simulink model "encoder_slsp"  (Simulink 8.0)
settings: Solver=FixedStepDiscrete  SolverMode=SingleTasking  StartTime=0.0  StopTime=10.0  RelTol=1e-3
settings Model: Creator=gcampa  LastModifiedBy=gcampa  ExtModeTrigDuration=2
settings DataIOCC: SignalLoggingSaveFormat=ModelDataLogs  SaveOutput=off  SaveTime=off
settings OptimizationCC: OptimizeModelRefInitCode=on  LifeSpan=1
settings DebuggingCC: SolverPrmCheckMsg=none  FcnCallInpInsideContextMsg=EnableAllAsWarning  StrictBusMsg=Warning
settings HardwareCC: ProdBitPerInt=16  ProdBitPerPointer=16  ProdIntDivRoundTo=Zero  ProdEndianess=LittleEndian  ProdWordSize=8  ProdHWDeviceType=Atmel->AVR
settings RTWCC: SystemTargetFile=realtime.tlc  GenerateMakefile=off  TemplateMakefile=realtime.tmf  Description=Real-Time Toolbox  RTWVerbose=off  ProcessScript=realtime_make_rtw_hook
settings STFCustomTargetCC: TargetLibSuffix=.a  CodeReplacementLibrary=ANSI_C  GenerateSampleERTMain=on  ERTCustomFileBanners=on  SupportNonInlinedSFcns=off  SupportVariableSizeSignals=on  GRTInterface=off  SystemTargetFile=realtime.tlc
settings ERTTargetCC: CodeReplacementLibrary=ANSI_C  MultiwordLength=2048  GenerateSampleERTMain=on  ParMdlRefBuildCompliant=off  CompOptLevelCompliant=off  ConcurrentExecutionCompliant=off  CombineOutputUpdateFcns=off  ERTFirstTimeCompliant=off  SupportContinuousTime=on  SupportVariableSizeSignals=on  ModelStepFunctionPrototypeControlCompliant=off  CPPClassGenCompliant=off  ExtModeTransport=3  ExtModeMexFile=ext_serial_win32_comm  ExtModeMexArgs=0 1 9600  InlinedParameterPlacement=NonHierarchical  ERTSrcFileBannerTemplate=realtime_code_template.cgt  ERTHdrFileBannerTemplate=realtime_code_template.cgt  ERTDataSrcFileTemplate=realtime_code_template.cgt  ERTDataHdrFileTemplate=realtime_code_template.cgt  ERTCustomFileTemplate=realtime_file_process.tlc  ConvertIfToSwitch=off  SuppressUnreachableDefaultCases=off
settings SettingsController: Description=Run on Hardware Dialog  TargetExtensionPlatform=Arduino Uno
settings MATStruct: Set_host_COM_port=[0.0]  COM_port_number=1  COM_port_baud_rate=115200  Enable_overrun_detection=[0.0]  Digital_output_to_set_on_overrun=13  Analog_input_reference_voltage=[0.0]  Serial0_baud_rate=115200

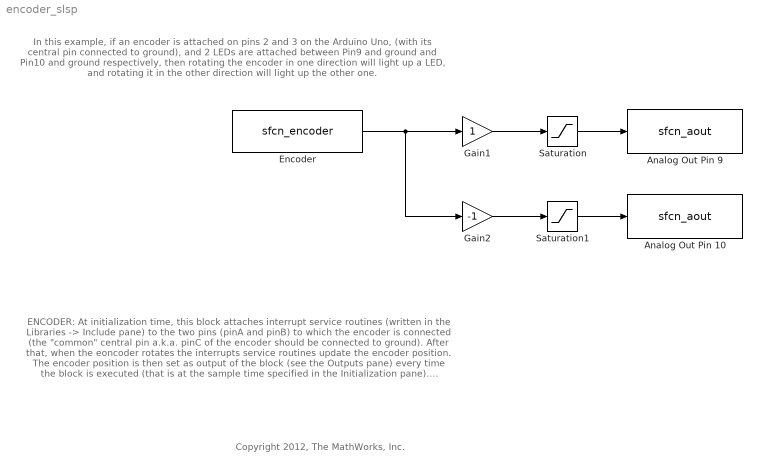
== system encoder_slsp ==
  note: In this example, if an encoder is attached on pins 2 and 3 on the Arduino Uno, (with its central pin connected to ground),
      | and 2 LEDs are attached between Pin9 and ground and Pin10 and ground respectively, then rotating the encoder in one
      | direction will light up a LED, and rotating it in the other direction will light up the other one.
  note: ENCODER: At initialization time, this block attaches interrupt service routines (written in the Libraries -> Include pane)
      |                     to the two pins (pinA and pinB) to which the encoder is connected (the "common" central pin a.k.a. pinC of
      |                     the encoder should be connected to ground).
      |                     After that, when the eoncoder rotates the interrupts service routines update the encoder position.
      |                     The encoder position is then set as output of the block (see the Outputs pane) every time the block is
      |                     executed (that is at the sample time specified in the Initialization pane).
      |
      | Parameters: enc is the encoder identifier, must be either 0, 1 or 2.
      |                      PinA and PinB are the pins to which the encoder is attached. The allowed pins are 2 and 3 on the uno board
      |                      and 2,3,18,19,20,21 on the mega board (see also http://arduino.cc/it/Reference/AttachInterrupt for details).
      |
      | Note that the encoder routines are the same as the ones used for the MATLAB Support Package for Arduino, so you might
      | also have a look at that package for additional explanations.
  note: Copyright 2012, The MathWorks, Inc.
  Analog Out Pin 10 : S-Function  InitFcn=try, set_param(gcb,'FunctionName','sfcn_aout'), end  FunctionName=sfcn_aout  Parameters=uint8(10)  SFunctionModules=sfcn_aout_wrapper  WizardData=DataTag0  EnableBusSupport=off  mask(S-Function Builder){}
      mask init:
      | val = [[.9  0.75 0.75 1 1 .9 .9 1]',[1 1 0.75 0.75 .9 .9 1 .9]'];try , sys = get_param(gcb,'SfunBuilderFcnName');if isempty(sys), sys = get_param(gcb,'FunctionName'); end,catch, sys = get_param(gcb,'FunctionName'); end
      settings: CopyFcn=set_param(gcbh,'LinkStatus','none')  PreSaveFcn=try, set_param(gcb,'FunctionName','sfcn_aout'), end  OpenFcn=sfunctionwizard(gcbh)
      mask Display: plot(val(:,1),val(:,2)),disp(sys), port_label('input',1,'in')
  Analog Out Pin 9 : S-Function  InitFcn=try, set_param(gcb,'FunctionName','sfcn_aout'), end  FunctionName=sfcn_aout  Parameters=uint8(9)  SFunctionModules=sfcn_aout_wrapper  WizardData=DataTag1  EnableBusSupport=off  mask(S-Function Builder){}
      mask init: same as encoder_slsp/Analog Out Pin 10
      settings: CopyFcn=set_param(gcbh,'LinkStatus','none')  PreSaveFcn=try, set_param(gcb,'FunctionName','sfcn_aout'), end  OpenFcn=sfunctionwizard(gcbh)
      mask Display: plot(val(:,1),val(:,2)),disp(sys), port_label('input',1,'in')
  Encoder : S-Function  InitFcn=try, set_param(gcb,'FunctionName','sfcn_encoder'), end  FunctionName=sfcn_encoder  Parameters=uint8(0),uint8(2),uint8(3)  SFunctionModules=sfcn_encoder_wrapper  WizardData=DataTag2  EnableBusSupport=off  mask(S-Function Builder){}
      mask init: same as encoder_slsp/Analog Out Pin 10
      settings: CopyFcn=set_param(gcbh,'LinkStatus','none')  PreSaveFcn=try, set_param(gcb,'FunctionName','sfcn_encoder'), end  OpenFcn=sfunctionwizard(gcbh)
      mask Display: plot(val(:,1),val(:,2)),disp(sys), port_label('output',1,'pos')
  Gain1 : Gain  OutDataTypeStr=Inherit: Same as input
  Gain2 : Gain  Gain=-1  OutDataTypeStr=Inherit: Same as input
  Saturation : Saturate  UpperLimit=255  LowerLimit=0  OutDataTypeStr=uint8
  Saturation1 : Saturate  UpperLimit=255  LowerLimit=0  OutDataTypeStr=uint8
  wires:
  Gain2/1 -> Saturation1/1
  Encoder/1 -> Gain2/1, Gain1/1
  Gain1/1 -> Saturation/1
  Saturation/1 -> Analog Out Pin 9/1
  Saturation1/1 -> Analog Out Pin 10/1
